simulink model "Tethermodel_R2018B"  (R2018b)
settings: Solver=FixedStepAuto  StartTime=0.0  StopTime=simInit.TSIM  FixedStep=simInit.dt  MaxStep=0.01  RelTol=1e-1
InitFcn:
  | close all
undefined symbols (not defined in the file or in its folder): DE2019, ENVMT, T
Description:
  | % Copyright 2020 Delft University of Technology
  | %
  | % Licensed under the Apache License, Version 2.0 (the "License");
  | % you may not use this file except in compliance with the License.
  | % You may obtain a copy of the License at
  | %
  | %      http://www.apache.org/licenses/LICENSE-2.0
  | %
  | % Unless required by applicable law or agreed to in writing, software
  | % distributed under the License is distributed on an "AS IS" BASIS,
  | % WITHOUT WARRANTIES OR CONDITIONS OF ANY KIND, either express or implied.
  | % See the License for the specific language governing permissions and
  | % limitations under the License.
settings Model: ExtModeTrigDuration=100  Creator=Sebastian  LastModifiedBy=dylaneijkelhof
settings SolverCC: SolverJacobianMethodControl=FullAnalytical
settings DataIOCC: SaveFormat=Array  SaveOutput=off  DSMLogging=off  SaveTime=off  StateSaveName=tmp_raccel_xout  SignalLoggingName=logged_signals  LoggingFileName=log
settings OptimizationCC: EfficientMapNaN2IntZero=off  LifeSpan=inf
settings DebuggingCC: ArtificialAlgebraicLoopMsg=none  SaveWithDisabledLinksMsg=none  SaveWithParameterizedLinksMsg=none  MaskedZcDiagnostic=none  IgnoredZcDiagnostic=none  InheritedTsInSrcMsg=none  TasksWithSamePriorityMsg=none  SigSpecEnsureSampleTimeMsg=none  ParameterPrecisionLossMsg=none  UnconnectedInputMsg=none  UnconnectedOutputMsg=none  UnconnectedLineMsg=none  BusObjectLabelMismatch=none  RootOutportRequireBusObject=none  UnknownTsInhSupMsg=none  ModelReferenceDataLoggingMessage=none  ModelReferenceSymbolNameMessage=none  InitInArrayFormatMsg=none  SFUnusedDataAndEventsDiag=none  SFUnexpectedBacktrackingDiag=none  SFInvalidInputDataAccessInChartInitDiag=none  SFNoUnconditionalDefaultTransitionDiag=none  SFTransitionOutsideNaturalParentDiag=none  SFUnreachableExecutionPathDiag=none  SFUndirectedBroadcastEventsDiag=none  SFTransitionActionBeforeConditionDiag=none  SFTemporalDelaySmallerThanSampleTimeDiag=none  SFSelfTransitionDiag=none  SFExecutionAtInitializationDiag=none  SFMachineParentedDataDiag=none  UnitsInconsistencyMsg=none
settings HardwareCC: TargetBitPerLong=64  TargetBitPerPointer=64  TargetBitPerSizeT=64  TargetBitPerPtrDiffT=64  TargetLongLongMode=on  TargetIntDivRoundTo=Zero  TargetEndianess=LittleEndian  TargetWordSize=64  TargetHWDeviceType=MATLAB Host  ProdEqTarget=off
settings ModelReferenceCC: PropagateSignalLabelsOutOfModel=off
settings SFSimCC: SimUseLocalCustomCode=off
settings CodeAppCC: MaxIdLength=128
settings GRTTargetCC: TargetLangStandard=C89/C90 (ANSI)  CombineOutputUpdateFcns=off  GRTInterface=on
settings ConfigComp: CovMetricSettings=dw  CovHtmlReporting=on  CovSaveCumulativeToWorkspaceVar=on  CovSaveSingleToWorkspaceVar=on  CovExternalEMLEnable=off

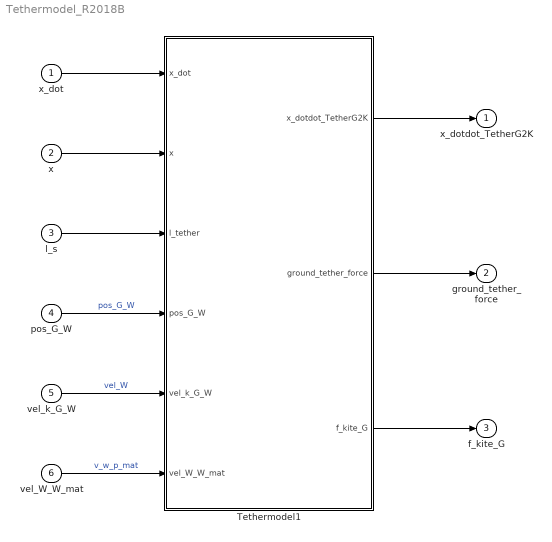
== system Tethermodel_R2018B ==
  x_dot : Inport  OutDataTypeStr=double
  x : Inport  Port=2  OutDataTypeStr=double
  l_s : Inport  Port=3  OutDataTypeStr=double  PortDimensions=1
  pos_G_W : Inport  Port=4  OutDataTypeStr=double  PortDimensions=[3,1]
  vel_k_G_W : Inport  Port=5  OutDataTypeStr=double  PortDimensions=[3,1]
  vel_W_W_mat : Inport  Port=6  OutDataTypeStr=double  PortDimensions=[3,T.np]
  Tethermodel1 : MATLAB Function  TreatAsAtomicUnit=on
  x_dotdot_TetherG2K : Outport  OutDataTypeStr=double  VectorParamsAs1DForOutWhenUnconnected=off
  ground_tether_force : Outport  Port=2  OutDataTypeStr=double  VectorParamsAs1DForOutWhenUnconnected=off
  f_kite_G : Outport  Port=3  OutDataTypeStr=double  VectorParamsAs1DForOutWhenUnconnected=off
  wires:
  x_dot/1 -> Tethermodel1/1(x_dot)
  x/1 -> Tethermodel1/2(x)
  l_s/1 -> Tethermodel1/3(l_tether)
  pos_G_W/1 -> Tethermodel1/4(pos_G_W)  "pos_G_W"
  vel_k_G_W/1 -> Tethermodel1/5(vel_k_G_W)  "vel_W"
  vel_W_W_mat/1 -> Tethermodel1/6(vel_W_W_mat)  "v_w_p_mat"
  Tethermodel1/1(x_dotdot_TetherG2K) -> x_dotdot_TetherG2K/1
  Tethermodel1/2(ground_tether_force) -> ground_tether_force/1
  Tethermodel1/3(f_kite_G) -> f_kite_G/1

== matlab function Tethermodel_R2018B/Tethermodel1 ==
  data: x_dot input size=[3*T.np,1]; x_dotdot_TetherG2K output size=[3*T.np,1]; x input size=[3*T.np,1]; l_tether input size=[1,1]; pos_G_W input; vel_k_G_W input; ground_tether_force output size=[3,1]; ENVMT parameter; T parameter; f_kite_G output size=[3,1]; vel_W_W_mat input; DE2019 parameter
% Copyright 2020 Delft University of Technology
%
% Licensed under the Apache License, Version 2.0 (the "License");
% you may not use this file except in compliance with the License.
% You may obtain a copy of the License at
%
%      http://www.apache.org/licenses/LICENSE-2.0
%
% Unless required by applicable law or agreed to in writing, software
% distributed under the License is distributed on an "AS IS" BASIS,
% WITHOUT WARRANTIES OR CONDITIONS OF ANY KIND, either express or implied.
% See the License for the specific language governing permissions and
% limitations under the License.

function [x_dotdot_TetherG2K, ground_tether_force,f_kite_G]    = pure_tether_model_function(x_dot, x,l_tether, pos_G_W,vel_k_G_W,ENVMT, T, vel_W_W_mat,DE2019)
%% Readme
% Equations are adapted from Fechner et al, Dynamic Model of a Pumping Kite
% Power System, Renewable Energy, 2015.
% Implementation: Sebastian Rapp, Wind Energy Institute, Faculty of
% Aerospace Engineering, TU Delft
% Mail: s.rapp@tudelft.nl
% Last change: 19.01.2018
%
% General description:
% This functions calculates the accelerations of the tether particle
% segment based on the acting forces at each particle.
%
% Inputs:
% x_dot: Tether particle velocities (world frame i.e. inertial frame)
% x: Tether particle position (world frame)
% v_w: wind vector (world frame)
% d_tether: tether diameter
% CD_tether: tether drag coefficient
% v_ro_set: reelout speed of the tether
% l_s: tether segment length
% c0: intial spring constant of a tether segment
% d0: initial damping constant of a tether segment
% rho_t: tether mass density (i.e. mass per m)
% g_vec: gravity vector
% rho_air: air density
% x_kite_A,C,D: position bridle attachment points
% xdot_kite_A,C,D: velocities of bridle attachment points
% ls_AKcu,CKcu,DKcu: bridle lengths
% m_kcu: kcu weight
%
% Outputs:
% x_dotdot_TetherG2K: accelertions of the tether particles
% l_s_dot: tether length increases with this speed
% ground_tether_force: tether force as measured at the ground

c0 = T.c0;
d0 = T.d0;
rho_t = DE2019.rho_tether;% T.rho_t; 
d_tether = DE2019.d_tether;%  T.d_tether;
CD_tether = DE2019.Cd_tether;% T.CD_tether;

n_t_p = T.np; % amount of particles
l_s = l_tether/(n_t_p+1); % Particle speeds

% Adapt stiffness and damping with respect to current segment length
% c = c0/max(l_s,60);
% d = d0/max(l_s,60);

c = c0/60; 
d = d0/60;

% Mass of tether segments with  respect to current segment length
m = l_s * rho_t;
m_vec = m * ones(n_t_p,1);
%m_vec(n_t_p) = (l_s/2 * rho_t);

p_vec = x;
v_vec = x_dot;
p_norm = zeros(n_t_p,1);

% Vector with distances between particles
p_d = p_vec - [0;0;0; p_vec(1:3*n_t_p-3)];

% Vector with velocity differences
v_d = v_vec - [0;0;0; v_vec(1:3*n_t_p-3)];
%v_d = v_vec - [p_d(1:3)*l_s_dot; v_vec(1:3*n_t_p-3)];

% calculate absolute distances between points
for iter = 1 : n_t_p
    p_norm(iter) = norm( p_d( (iter-1)* 3 + 1 : (iter-1) * 3 + 3 ) );
end

% Gravity vector in W frame
g_vec = [0;0;ENVMT.g];

%%------------------------------- Set up equations of motion-------------------------------
% Initialize matrices
fsd_tot_mat = zeros(3,n_t_p);
x_dotdot = zeros(3,n_t_p);
D_s_mat = zeros(3,n_t_p);

%% Set up equations of motions of ground to kite tether

% Boundary tether force from kite to particle below kite (in the 4p kite model the kcu is connected to the
% points A, C and D

f_kite_G = calcSpringDamperForce( c0,norm( pos_G_W - p_vec(3*(n_t_p) -2 : 3*(n_t_p) ) ), l_s, d0,...
    pos_G_W - p_vec(3*(n_t_p) -2 : 3*(n_t_p) ) ,...
    vel_k_G_W - v_vec( 3*(n_t_p) -2 : 3*(n_t_p)  ) );

v_a_p_save = zeros(3, n_t_p);

% Loop through all particles
for idx = 1 : n_t_p
    v_w_vec = vel_W_W_mat(:,idx);
    % Calculate Spring-Damper forces
    fsd_tot_mat(:,idx) = calcSpringDamperForce( c, p_norm(idx), l_s, d, p_d( (idx-1)*3+1:(idx-1)*3+3 ), v_d( (idx-1)*3+1:(idx-1)*3+3) );
    if idx < n_t_p
        fsd_tot_mat(:,idx+1) = calcSpringDamperForce( c, p_norm(idx+1), l_s, d, p_d( idx*3+1:idx*3+3 ), v_d( idx*3+1:idx*3+3) );
    end
    
    % Calculate apparent wind speed of tether particles
    if idx == 1 % Segment that is connected to the ground
        v_a_p = v_w_vec - 0.5*x_dot(1:3) ;
    elseif idx == n_t_p
        v_a_p = v_w_vec - 0.5*( x_dot((idx-2)*3+1:(idx-2)*3+3) + x_dot( (idx-1)*3+1:(idx-1)*3+3) ); % take mean value of adjacent particle vel. for segment velocity
    else
        v_a_p = v_w_vec - 0.5*( x_dot((idx-2)*3+1:(idx-2)*3+3) + x_dot( (idx-1)*3+1:(idx-1)*3+3) ); % take mean value of adjacent particle vel. for segment velocity
    end
    v_a_p_save(1:3, idx) = v_a_p;
    
    % Calculate segment drag
    D_s_mat(:,idx) = 1*calcSegmentDrag(p_d((idx-1)*3+1:(idx-1)*3+3) , v_a_p, ENVMT.rhos, CD_tether, d_tether); % segment drag
    if idx < n_t_p
        % Equations of motion for the groud tether particles Newton x_dotdot = 1/m * (-f + u -mg )
        if idx+1 == n_t_p
            x_dotdot(:,idx) = 1/m_vec(idx) * ( -fsd_tot_mat(:,idx) + 1*fsd_tot_mat(:,idx+1) - m_vec(idx)*g_vec  + D_s_mat(:,idx) );  % Particle dynamics
        else
            if idx == 1
                x_dotdot(:,idx) = 1/m_vec(idx) * ( -fsd_tot_mat(:,1) + fsd_tot_mat(:,2) - m_vec(1)*g_vec  + D_s_mat(:,1) );  % Particle dynamics
            else
                x_dotdot(:,idx) = 1/m_vec(idx) * ( -fsd_tot_mat(:,idx) + 1*fsd_tot_mat(:,idx+1) - m_vec(idx)*g_vec  + D_s_mat(:,idx) );  % Particle dynamics
            end
        end
    else
        % Flexible tether: last particle of the tether is connected to the aircraft CG.
        x_dotdot(:,idx) = 1/m_vec(idx) * ( -1*fsd_tot_mat(:,idx) + f_kite_G - m_vec(idx)*g_vec  + D_s_mat(:,idx) );  % Particle dynamics
    end
    
    ground_tether_force =  fsd_tot_mat(:,1);
    
end

x_dotdot_TetherG2K = reshape(x_dotdot, [3*n_t_p,1]);

end
